simulink model "proj7_week1"  (R2020b)
settings: Solver=VariableStepAuto  StartTime=0.0  StopTime=10.0  RelTol=1e-3
settings Model: Creator=RASIKA MALGI  LastModifiedBy=RASIKA MALGI

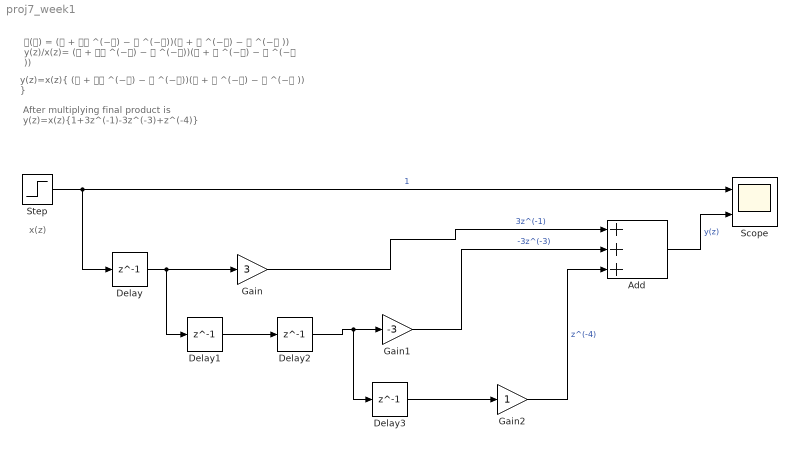
== system proj7_week1 ==
  note: After multiplying final product is
      | y(z)=x(z){1+3z^(-1)-3z^(-3)+z^(-4)}
  note: y(z)=x(z){ (𝟏 + 𝟐𝐳 ^(−𝟏) − 𝐳 ^(−𝟐))(𝟏 + 𝐳 ^(−𝟏) − 𝐳 ^(−𝟐 )) }
  note: 𝐇(𝐳) = (𝟏 + 𝟐𝐳 ^(−𝟏) − 𝐳 ^(−𝟐))(𝟏 + 𝐳 ^(−𝟏) − 𝐳 ^(−𝟐 ))
      | y(z)/x(z)= (𝟏 + 𝟐𝐳 ^(−𝟏) − 𝐳 ^(−𝟐))(𝟏 + 𝐳 ^(−𝟏) − 𝐳 ^(−𝟐 ))
  note: x(z)
  Add : Sum  Inputs=+++
  Delay{,1..3} (4 alike) : Delay  DelayLength=1  InitialCondition=0
  Gain : Gain  Gain=3
  Gain1 : Gain  Gain=-3
  Gain2 : Gain
  Scope : Scope  NumInputPorts=2
  Step : Step  SampleTime=0
  wires:
  Delay/1 -> Delay1/1, Gain/1
  Step/1 -> Scope/1, Delay/1  "1"
  Delay1/1 -> Delay2/1
  Delay2/1 -> Delay3/1, Gain1/1
  Delay3/1 -> Gain2/1
  Gain/1 -> Add/1  "3z^(-1)"
  Gain1/1 -> Add/2  "-3z^(-3)"
  Gain2/1 -> Add/3  "z^(-4)"
  Add/1 -> Scope/2  "y(z)"
